simulink model "Asw_DCAC"  (R2023b)
settings: Solver=FixedStepDiscrete  StartTime=0.0  StopTime=inf  FixedStep=1e-8  RelTol=1e-3  EnableMultiTasking=on
undefined symbols (not defined in the file): f_Vref, Ts, V_DC
libraries: slpidlib x5, simulink x1
settings Model: Creator=VanillaC  LastModifiedBy=VanillaC
settings OptimizationCC: DefaultParameterBehavior=Inlined  EnhancedBackFolding=on  PassReuseOutputArgsAs=Individual arguments  ZeroExternalMemoryAtStartup=off  ZeroInternalMemoryAtStartup=off  MaxStackSize=64  OptimizeBlockOrder=speed  DifferentSizesBufferReuse=on  OptimizationCustomize=off  EfficientTunableParamExpr=on
settings DebuggingCC: ParameterTunabilityLossMsg=error
settings HardwareCC: ProdBitPerPointer=32  ProdBitPerSizeT=32  ProdBitPerPtrDiffT=32  ProdLargestAtomicInteger=Long  ProdLargestAtomicFloat=Double  ProdWordSize=32  ProdHWDeviceType=ARM Compatible->ARM Cortex-M
settings SFSimCC: MATLABDynamicMemAlloc=off
settings RTWCC: Description=Embedded Coder  SystemTargetFile=ert.tlc  GenCodeOnly=on  TemplateMakefile=ert_default_tmf  Toolchain=GNU Tools for ARM Embedded Processors
settings CodeAppCC: ForceParamTrailComments=on  IgnoreCustomStorageClasses=off  OperatorAnnotations=on  SimulinkDataObjDesc=on  SFDataObjDesc=on  InsertBlockDesc=on
settings ERTTargetCC: TargetLangStandard=C99 (ISO)  CodeReplacementLibrary=ARM Cortex-M  ExtModeTransport=3  ExtModeStaticAlloc=on  ExtModeStaticAllocSize=2048  ExtModeMexFile=ext_xcp  ExtModeIntrfLevel=Level2 - Open  InlinedParameterPlacement=NonHierarchical  ERTCustomFileTemplate=example_file_process.tlc

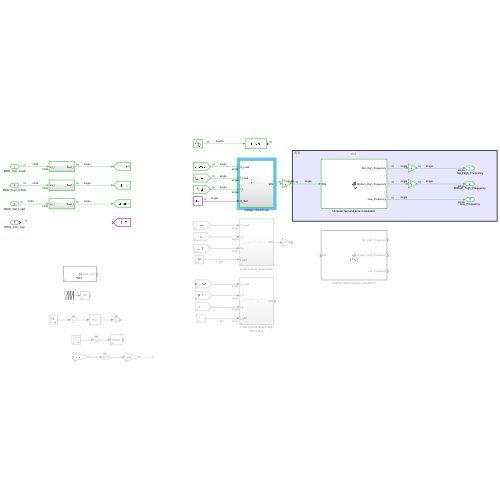
[thumbnail: Simulink's stored preview of the top-level diagram]
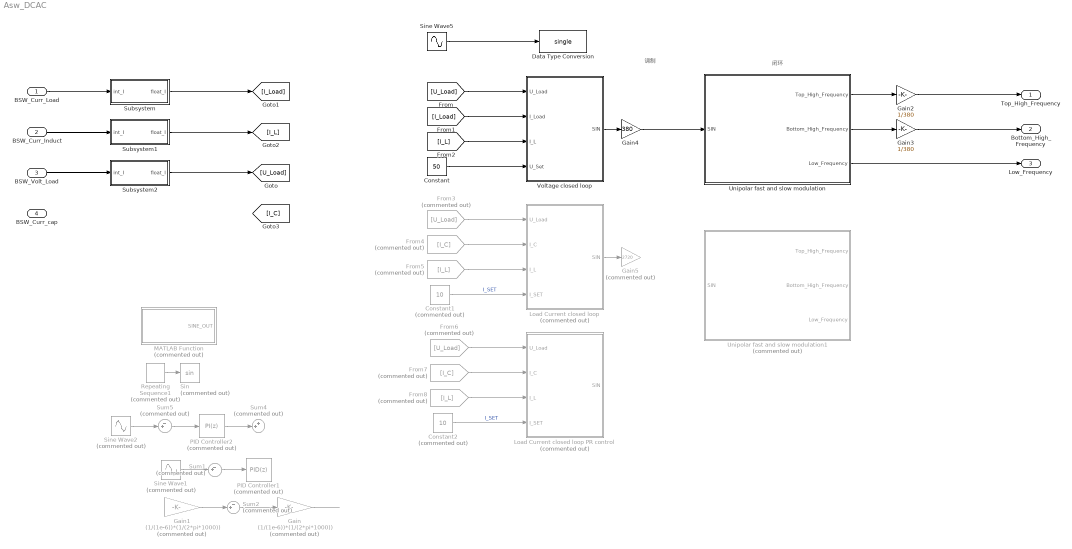
== system Asw_DCAC ==
  note: 闭环
  note: 调制
  BSW_Curr_Load : Inport  OutDataTypeStr=int32
  BSW_Curr_Induct : Inport  Port=2  OutDataTypeStr=int32
  BSW_Volt_Load : Inport  Port=3  OutDataTypeStr=int32
  BSW_Curr_cap : Inport  Port=4  OutDataTypeStr=single
  Constant : Constant  Value=50  OutDataTypeStr=single
  Constant1 : Constant  Commented=on  Value=10  OutDataTypeStr=single
  Constant2 : Constant  Commented=on  Value=10  OutDataTypeStr=single
  Data Type Conversion : DataTypeConversion  OutDataTypeStr=single  SaturateOnIntegerOverflow=off  RndMeth=Floor
  From3 : From  Commented=on  GotoTag=U_Load
  From4 : From  Commented=on  GotoTag=I_C
  From5 : From  Commented=on  GotoTag=I_L
  From6 : From  Commented=on  GotoTag=U_Load
  From7 : From  Commented=on  GotoTag=I_C
  From8 : From  Commented=on  GotoTag=I_L
  Gain : Gain  Commented=on  Gain=(1/(1e-6))*(1/(2*pi*1000))  OutDataTypeStr=single
  Gain1 : Gain  Commented=on  Gain=(1/(1e-6))*(1/(2*pi*1000))  OutDataTypeStr=single
  Gain2 : Gain  Gain=1/380
  Gain3 : Gain  Gain=1/380
  Gain4 : Gain  Gain=380
  Gain5 : Gain  Commented=on  Gain=2720
  Load Current closed loop : Subsystem  Commented=on
  Load Current closed loop PR control : Subsystem  Commented=on
  MATLAB Function : MATLAB Function  Commented=on  TreatAsAtomicUnit=on
  PID Controller1 : slpidlib/PID Controller  Commented=on  Controller=PID  Form=Parallel  TimeDomain=Discrete-time  UseExternalTs=off  SampleTime=-1  IntegratorMethod=Trapezoidal  FilterMethod=Forward Euler  ControllerParametersSource=internal  P=0.5  I=0.5  UseKiTs=off  D=0  N=100  UseFilter=off  TunerSelectOption=Transfer Function Based (PID Tuner App)  InitialConditionSource=internal  InitialConditionForIntegrator=0  InitialConditionForFilter=0  DifferentiatorICPrevScaledInput=0  ExternalReset=none  TrackingMode=off  Kt=1  LimitOutput=off  SatLimitsSource=internal  UpperSaturationLimit=inf  LowerSaturationLimit=-inf  LinearizeAsGain=on  AntiWindupMode=none  Kb=1  LimitIntegrator=off  UpperIntegratorSaturationLimit=inf  LowerIntegratorSaturationLimit=-inf  POutMin=[]  POutMax=[]  IOutMin=[]  IOutMax=[]  DOutMin=[]  DOutMax=[]  NOutMin=[]  NOutMax=[]  SumOutMin=[]  SumOutMax=[]  SaturationOutMin=[]  SaturationOutMax=[]  PParamMin=[]  PParamMax=[]  IParamMin=[]  IParamMax=[]  DParamMin=[]  DParamMax=[]  NParamMin=[]  NParamMax=[]  KbParamMin=[]  KbParamMax=[]  KtParamMin=[]  KtParamMax=[]  KbOutMin=[]  KbOutMax=[]  KtOutMin=[]  KtOutMax=[]  IntegratorOutMin=[]  IntegratorOutMax=[]  FilterOutMin=[]  FilterOutMax=[]  SumI1OutMin=[]  SumI1OutMax=[]  SumI2OutMin=[]  SumI2OutMax=[]  SumI3OutMin=[]  SumI3OutMax=[]  SumI4OutMin=[]  SumI4OutMax=[]  SumDOutMin=[]  SumDOutMax=[]  DifferentiatorOutMin=[]  DifferentiatorOutMax=[]  FilterDiffOutCoefMin=[]  FilterDiffOutCoefMax=[]  ReciprocalOutMin=[]  ReciprocalOutMax=[]  SumDenOutMin=[]  SumDenOutMax=[]  SumNumOutMin=[]  SumNumOutMax=[]  DivideOutMin=[]  DivideOutMax=[]  UdiffTsProdOutMin=[]  UdiffTsProdOutMax=[]  NTsProdOutMin=[]  NTsProdOutMax=[]  UintegralTsProdOutMin=[]  UintegralTsProdOutMax=[]  UngainTsProdOutMin=[]  UngainTsProdOutMax=[]  ClampingZeroOutDataTypeStr=Inherit: Inherit via back propagation  ClampingZeroOutMin=[]  ClampingZeroOutMax=[]  FilterDenConstantOutDataTypeStr=Inherit: Inherit via back propagation  FilterDenConstantOutMin=[]  FilterDenConstantOutMax=[]  PCopyOutDataTypeStr=Inherit: Inherit via back propagation  PCopyOutMin=[]  PCopyOutMax=[]  NCopyOutDataTypeStr=Inherit: Inherit via back propagation  NCopyOutMin=[]  NCopyOutMax=[]  IntegratorContinuousStateAttributes=''  IntegratorStateMustResolveToSignalObject=off  IntegratorRTWStateStorageClass=Auto  FilterContinuousStateAttributes=''  FilterStateMustResolveToSignalObject=off  FilterRTWStateStorageClass=Auto  ParallelPVariant=InternalParameters  IdealPVariant=Disabled  IVariant=InternalParameters  DVariant=InternalParameters  IntegratorVariant=Discrete  SatVariant=Disabled  AWVariant=Passthrough  PCopyVariant=Disabled  TRVariant=Disabled  FdbkBlocksVariant=Forward  IdealPFdbkVariant=Disabled  SatFdbkVariant=Disabled  DerivativeFilterVariant=Differentiator  NVariant=Passthrough  NCopyVariant=Disabled_SignalSpec  FilterICVariant=InternalICsDifferentiator  IntegratorICVariant=InternalICs  ExternalResetVariant=Disabled  TRSumVariant=Passthrough  SumFdbkVariant=Disabled  SumVariant=Sum_PID  TsampFilterVariant=InternalTs  TsampNgainVariant=Passthrough  TsampIntegralVariant=Disabled_SignalSpec  ExternalSaturationOutDataTypeStr=Inherit: Same as second input
  PID Controller2 : slpidlib/PID Controller  Commented=on  Controller=PI  Form=Parallel  TimeDomain=Discrete-time  UseExternalTs=off  SampleTime=-1  IntegratorMethod=Trapezoidal  FilterMethod=Forward Euler  ControllerParametersSource=internal  P=0.05115  I=30  UseKiTs=off  D=0  N=100  UseFilter=off  TunerSelectOption=Transfer Function Based (PID Tuner App)  InitialConditionSource=internal  InitialConditionForIntegrator=0  InitialConditionForFilter=0  DifferentiatorICPrevScaledInput=0  ExternalReset=none  TrackingMode=off  Kt=1  LimitOutput=off  SatLimitsSource=internal  UpperSaturationLimit=inf  LowerSaturationLimit=-inf  LinearizeAsGain=on  AntiWindupMode=none  Kb=1  LimitIntegrator=off  UpperIntegratorSaturationLimit=inf  LowerIntegratorSaturationLimit=-inf  POutMin=[]  POutMax=[]  IOutMin=[]  IOutMax=[]  DOutMin=[]  DOutMax=[]  NOutMin=[]  NOutMax=[]  SumOutMin=[]  SumOutMax=[]  SaturationOutMin=[]  SaturationOutMax=[]  PParamMin=[]  PParamMax=[]  IParamMin=[]  IParamMax=[]  DParamMin=[]  DParamMax=[]  NParamMin=[]  NParamMax=[]  KbParamMin=[]  KbParamMax=[]  KtParamMin=[]  KtParamMax=[]  KbOutMin=[]  KbOutMax=[]  KtOutMin=[]  KtOutMax=[]  IntegratorOutMin=[]  IntegratorOutMax=[]  FilterOutMin=[]  FilterOutMax=[]  SumI1OutMin=[]  SumI1OutMax=[]  SumI2OutMin=[]  SumI2OutMax=[]  SumI3OutMin=[]  SumI3OutMax=[]  SumI4OutMin=[]  SumI4OutMax=[]  SumDOutMin=[]  SumDOutMax=[]  DifferentiatorOutMin=[]  DifferentiatorOutMax=[]  FilterDiffOutCoefMin=[]  FilterDiffOutCoefMax=[]  ReciprocalOutMin=[]  ReciprocalOutMax=[]  SumDenOutMin=[]  SumDenOutMax=[]  SumNumOutMin=[]  SumNumOutMax=[]  DivideOutMin=[]  DivideOutMax=[]  UdiffTsProdOutMin=[]  UdiffTsProdOutMax=[]  NTsProdOutMin=[]  NTsProdOutMax=[]  UintegralTsProdOutMin=[]  UintegralTsProdOutMax=[]  UngainTsProdOutMin=[]  UngainTsProdOutMax=[]  ClampingZeroOutDataTypeStr=Inherit: Inherit via back propagation  ClampingZeroOutMin=[]  ClampingZeroOutMax=[]  FilterDenConstantOutDataTypeStr=Inherit: Inherit via back propagation  FilterDenConstantOutMin=[]  FilterDenConstantOutMax=[]  PCopyOutDataTypeStr=Inherit: Inherit via back propagation  PCopyOutMin=[]  PCopyOutMax=[]  NCopyOutDataTypeStr=Inherit: Inherit via back propagation  NCopyOutMin=[]  NCopyOutMax=[]  IntegratorContinuousStateAttributes=''  IntegratorStateMustResolveToSignalObject=off  IntegratorRTWStateStorageClass=Auto  FilterContinuousStateAttributes=''  FilterStateMustResolveToSignalObject=off  FilterRTWStateStorageClass=Auto  ParallelPVariant=InternalParameters  IdealPVariant=Disabled  IVariant=InternalParameters  DVariant=Disabled  IntegratorVariant=Discrete  SatVariant=Disabled  AWVariant=Passthrough  PCopyVariant=Disabled  TRVariant=Disabled  FdbkBlocksVariant=Forward  IdealPFdbkVariant=Disabled  SatFdbkVariant=Disabled  DerivativeFilterVariant=Disabled  NVariant=Disabled  NCopyVariant=Disabled_SignalSpec  FilterICVariant=Disabled  IntegratorICVariant=InternalICs  ExternalResetVariant=Disabled  TRSumVariant=Passthrough  SumFdbkVariant=Disabled  SumVariant=Sum_PI  TsampFilterVariant=InternalTs  TsampNgainVariant=Passthrough  TsampIntegralVariant=Disabled_SignalSpec  ExternalSaturationOutDataTypeStr=Inherit: Same as second input
  Repeating Sequence1 : simulink/Sources/Repeating Sequence  Commented=on  rep_seq_t=[0 1/1000]  rep_seq_y=[0 2*pi]
  Sin : Trigonometry  Commented=on
  Sine Wave1 : Sin  Commented=on  Frequency=2*pi*1000  SampleTime=Ts
  Sine Wave2 : Sin  Commented=on  Amplitude=311  Frequency=f_Vref  SampleTime=Ts
  Sine Wave5 : Sin  Frequency=2*pi*1000  SampleTime=Ts
  Subsystem : Subsystem
  Subsystem1 : Subsystem
  Subsystem2 : Subsystem
  Sum1 : Sum  Commented=on  Inputs=-+|  OutDataTypeStr=single
  Sum2 : Sum  Commented=on  Inputs=-+|  OutDataTypeStr=single
  Sum4 : Sum  Commented=on  Inputs=++|
  Sum5 : Sum  Commented=on  Inputs=-+|  OutDataTypeStr=single
  Unipolar fast and slow modulation : MATLAB Function  TreatAsAtomicUnit=on
  Unipolar fast and slow modulation1 : MATLAB Function  Commented=on  TreatAsAtomicUnit=on
  Voltage closed loop : Subsystem
  Top_High_Frequency : Outport  OutDataTypeStr=single
  Bottom_High_Frequency : Outport  Port=2  OutDataTypeStr=single
  Low_Frequency : Outport  Port=3  OutDataTypeStr=single
  wires:
  Unipolar fast and slow modulation/2(Bottom_High_Frequency) -> Gain3/1
  Unipolar fast and slow modulation/1(Top_High_Frequency) -> Gain2/1
  Sum5/1 -> PID Controller2/1
  Sine Wave1/1 -> Sum1/2
  Sum1/1 -> PID Controller1/1
  Sine Wave5/1 -> Data Type Conversion/1
  Gain/1 -> ?
  Gain1/1 -> Sum2/2
  Sum2/1 -> Gain/1
  Sine Wave2/1 -> Sum5/2
  PID Controller2/1 -> Sum4/2
  Repeating Sequence1/1 -> Sin/1
  Constant/1 -> Voltage closed loop/4(U_Set)
  Constant1/1 -> Load Current closed loop/4(I_SET)  "I_SET"
  From5/1 -> Load Current closed loop/3(I_L)
  From4/1 -> Load Current closed loop/2(I_C)
  From3/1 -> Load Current closed loop/1(U_Load)
  [U_Load] -> Voltage closed loop/1(U_Load)
  [I_Load] -> Voltage closed loop/2(I_Load)
  [I_L] -> Voltage closed loop/3(I_L)
  From7/1 -> Load Current closed loop PR control/2(I_C)
  Constant2/1 -> Load Current closed loop PR control/4(I_SET)  "I_SET"
  From6/1 -> Load Current closed loop PR control/1(U_Load)
  From8/1 -> Load Current closed loop PR control/3(I_L)
  Gain2/1 -> Top_High_Frequency/1
  Gain3/1 -> Bottom_High_Frequency/1
  Unipolar fast and slow modulation/3(Low_Frequency) -> Low_Frequency/1
  Load Current closed loop/1(SIN) -> Gain5/1
  BSW_Curr_Load/1 -> Subsystem/1(int_I)
  BSW_Curr_Induct/1 -> Subsystem1/1(int_I)
  BSW_Volt_Load/1 -> Subsystem2/1(int_I)
  Subsystem/1(float_I) -> [I_Load]
  Subsystem1/1(float_I) -> [I_L]
  Subsystem2/1(float_I) -> [U_Load]
  Gain4/1 -> Unipolar fast and slow modulation/1(SIN)
  Voltage closed loop/1(SIN) -> Gain4/1

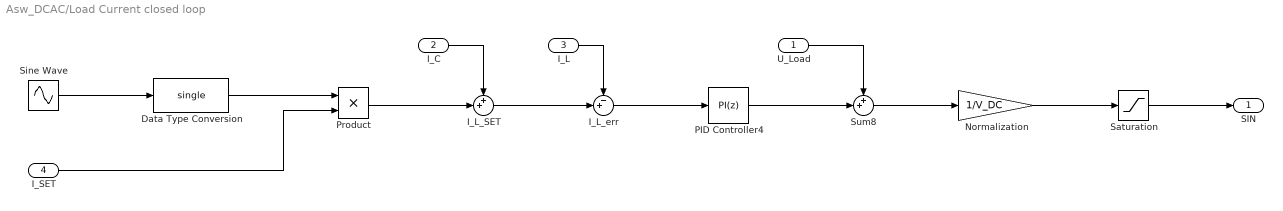
== system Asw_DCAC/Load Current closed loop ==
  U_Load : Inport  OutDataTypeStr=single
  I_C : Inport  Port=2  OutDataTypeStr=single
  I_L : Inport  Port=3  OutDataTypeStr=single
  I_SET : Inport  Port=4
  Data Type Conversion : DataTypeConversion  OutDataTypeStr=single  SaturateOnIntegerOverflow=off  RndMeth=Floor
  I_L_SET : Sum  Inputs=++|  OutDataTypeStr=single
  I_L_err : Sum  Inputs=-+|  OutDataTypeStr=single
  Normalization : Gain  Gain=1/V_DC  OutDataTypeStr=single
  PID Controller4 : slpidlib/PID Controller  Controller=PI  Form=Parallel  TimeDomain=Discrete-time  UseExternalTs=off  SampleTime=Ts  IntegratorMethod=Trapezoidal  FilterMethod=Forward Euler  ControllerParametersSource=internal  P=5  I=1  UseKiTs=off  D=0  N=100  UseFilter=off  TunerSelectOption=Transfer Function Based (PID Tuner App)  InitialConditionSource=internal  InitialConditionForIntegrator=0  InitialConditionForFilter=0  DifferentiatorICPrevScaledInput=0  ExternalReset=none  TrackingMode=off  Kt=1  LimitOutput=off  SatLimitsSource=internal  UpperSaturationLimit=inf  LowerSaturationLimit=-inf  LinearizeAsGain=on  AntiWindupMode=none  Kb=1  LimitIntegrator=off  UpperIntegratorSaturationLimit=inf  LowerIntegratorSaturationLimit=-inf  POutMin=[]  POutMax=[]  IOutMin=[]  IOutMax=[]  DOutMin=[]  DOutMax=[]  NOutMin=[]  NOutMax=[]  SumOutMin=[]  SumOutMax=[]  SaturationOutMin=[]  SaturationOutMax=[]  PParamMin=[]  PParamMax=[]  IParamMin=[]  IParamMax=[]  DParamMin=[]  DParamMax=[]  NParamMin=[]  NParamMax=[]  KbParamMin=[]  KbParamMax=[]  KtParamMin=[]  KtParamMax=[]  KbOutMin=[]  KbOutMax=[]  KtOutMin=[]  KtOutMax=[]  IntegratorOutMin=[]  IntegratorOutMax=[]  FilterOutMin=[]  FilterOutMax=[]  SumI1OutMin=[]  SumI1OutMax=[]  SumI2OutMin=[]  SumI2OutMax=[]  SumI3OutMin=[]  SumI3OutMax=[]  SumI4OutMin=[]  SumI4OutMax=[]  SumDOutMin=[]  SumDOutMax=[]  DifferentiatorOutMin=[]  DifferentiatorOutMax=[]  FilterDiffOutCoefMin=[]  FilterDiffOutCoefMax=[]  ReciprocalOutMin=[]  ReciprocalOutMax=[]  SumDenOutMin=[]  SumDenOutMax=[]  SumNumOutMin=[]  SumNumOutMax=[]  DivideOutMin=[]  DivideOutMax=[]  UdiffTsProdOutMin=[]  UdiffTsProdOutMax=[]  NTsProdOutMin=[]  NTsProdOutMax=[]  UintegralTsProdOutMin=[]  UintegralTsProdOutMax=[]  UngainTsProdOutMin=[]  UngainTsProdOutMax=[]  ClampingZeroOutDataTypeStr=Inherit: Inherit via back propagation  ClampingZeroOutMin=[]  ClampingZeroOutMax=[]  FilterDenConstantOutDataTypeStr=Inherit: Inherit via back propagation  FilterDenConstantOutMin=[]  FilterDenConstantOutMax=[]  PCopyOutDataTypeStr=Inherit: Inherit via back propagation  PCopyOutMin=[]  PCopyOutMax=[]  NCopyOutDataTypeStr=Inherit: Inherit via back propagation  NCopyOutMin=[]  NCopyOutMax=[]  IntegratorContinuousStateAttributes=''  IntegratorStateMustResolveToSignalObject=off  IntegratorRTWStateStorageClass=Auto  FilterContinuousStateAttributes=''  FilterStateMustResolveToSignalObject=off  FilterRTWStateStorageClass=Auto  ParallelPVariant=InternalParameters  IdealPVariant=Disabled  IVariant=InternalParameters  DVariant=Disabled  IntegratorVariant=Discrete  SatVariant=Disabled  AWVariant=Passthrough  PCopyVariant=Disabled  TRVariant=Disabled  FdbkBlocksVariant=Forward  IdealPFdbkVariant=Disabled  SatFdbkVariant=Disabled  DerivativeFilterVariant=Disabled  NVariant=Disabled  NCopyVariant=Disabled_SignalSpec  FilterICVariant=Disabled  IntegratorICVariant=InternalICs  ExternalResetVariant=Disabled  TRSumVariant=Passthrough  SumFdbkVariant=Disabled  SumVariant=Sum_PI  TsampFilterVariant=InternalTs  TsampNgainVariant=Passthrough  TsampIntegralVariant=Disabled_SignalSpec  ExternalSaturationOutDataTypeStr=Inherit: Same as second input
  Product : Product  OutDataTypeStr=single
  Saturation : Saturate  UpperLimit=1  LowerLimit=-1  OutDataTypeStr=single
  Sine Wave : Sin  Frequency=2*pi*1000  SampleTime=Ts
  Sum8 : Sum  Inputs=++|  OutDataTypeStr=single
  SIN : Outport
  wires:
  I_L_err/1 -> PID Controller4/1
  PID Controller4/1 -> Sum8/2
  Sine Wave/1 -> Data Type Conversion/1
  Data Type Conversion/1 -> Product/1
  I_L/1 -> I_L_err/1
  Sum8/1 -> Normalization/1
  Saturation/1 -> SIN/1
  I_SET/1 -> Product/2
  Normalization/1 -> Saturation/1
  U_Load/1 -> Sum8/1
  Product/1 -> I_L_SET/2
  I_L_SET/1 -> I_L_err/2
  I_C/1 -> I_L_SET/1

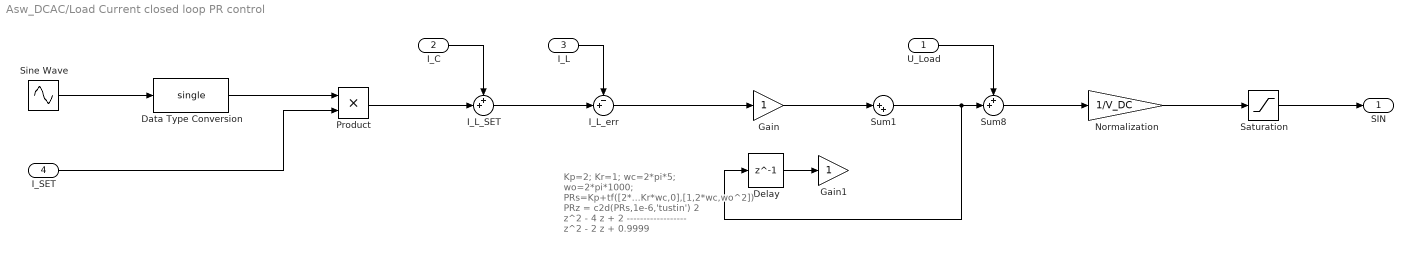
== system Asw_DCAC/Load Current closed loop PR control ==
  note: Kp=2; Kr=1; wc=2*pi*5; wo=2*pi*1000; PRs=Kp+tf([2*Kr*wc,0],[1,2*wc,wo^2]) PRz = c2d(PRs,1e-6,'tustin')
      |
      |  2 z^2 - 4 z + 2
      |   ------------------
      |   z^2 - 2 z + 0.9999
  U_Load : Inport  OutDataTypeStr=single
  I_C : Inport  Port=2  OutDataTypeStr=single
  I_L : Inport  Port=3  OutDataTypeStr=single
  I_SET : Inport  Port=4  OutDataTypeStr=single
  Data Type Conversion : DataTypeConversion  OutDataTypeStr=single  SaturateOnIntegerOverflow=off  RndMeth=Floor
  Delay : Delay  DelayLength=1
  Gain : Gain  OutDataTypeStr=single
  Gain1 : Gain  OutDataTypeStr=single
  I_L_SET : Sum  Inputs=++|  OutDataTypeStr=single
  I_L_err : Sum  Inputs=-+|  OutDataTypeStr=single
  Normalization : Gain  Gain=1/V_DC  OutDataTypeStr=single
  Product : Product  OutDataTypeStr=single
  Saturation : Saturate  UpperLimit=1  LowerLimit=-1  OutDataTypeStr=single
  Sine Wave : Sin  Frequency=2*pi*1000  SampleTime=Ts
  Sum1 : Sum  Inputs=|++  OutDataTypeStr=single
  Sum8 : Sum  Inputs=++|  OutDataTypeStr=single
  SIN : Outport
  wires:
  Sine Wave/1 -> Data Type Conversion/1
  Data Type Conversion/1 -> Product/1
  I_L/1 -> I_L_err/1
  Sum8/1 -> Normalization/1
  Saturation/1 -> SIN/1
  I_SET/1 -> Product/2
  Normalization/1 -> Saturation/1
  U_Load/1 -> Sum8/1
  Product/1 -> I_L_SET/2
  I_L_SET/1 -> I_L_err/2
  I_C/1 -> I_L_SET/1
  Gain/1 -> Sum1/1
  Delay/1 -> Gain1/1
  Sum1/1 -> Delay/1, Sum8/2
  I_L_err/1 -> Gain/1

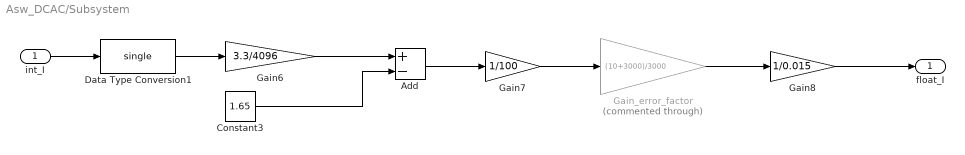
== system Asw_DCAC/Subsystem ==
  int_I : Inport  OutDataTypeStr=int32
  Add : Sum  Inputs=+-  OutDataTypeStr=single
  Constant3 : Constant  Value=1.65  OutDataTypeStr=single  SampleTime=-1
  Data Type Conversion1 : DataTypeConversion  OutDataTypeStr=single  SaturateOnIntegerOverflow=off  RndMeth=Floor
  Gain6 : Gain  Gain=3.3/4096  OutDataTypeStr=single
  Gain7 : Gain  Gain=1/100  OutDataTypeStr=single
  Gain8 : Gain  Gain=1/0.015  OutDataTypeStr=single
  Gain_error_factor : Gain  Commented=through  Gain=(10+3000)/3000  OutDataTypeStr=single
  float_I : Outport
  wires:
  Gain_error_factor/1 -> Gain8/1
  Constant3/1 -> Add/2
  Gain6/1 -> Add/1
  Gain7/1 -> Gain_error_factor/1
  Gain8/1 -> float_I/1
  int_I/1 -> Data Type Conversion1/1
  Data Type Conversion1/1 -> Gain6/1
  Add/1 -> Gain7/1

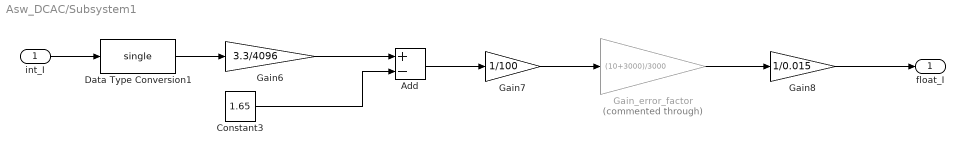
== system Asw_DCAC/Subsystem1 ==
  int_I : Inport  OutDataTypeStr=int32
  Add : Sum  Inputs=+-  OutDataTypeStr=single
  Constant3 : Constant  Value=1.65  OutDataTypeStr=single  SampleTime=-1
  Data Type Conversion1 : DataTypeConversion  OutDataTypeStr=single  SaturateOnIntegerOverflow=off  RndMeth=Floor
  Gain6 : Gain  Gain=3.3/4096  OutDataTypeStr=single
  Gain7 : Gain  Gain=1/100  OutDataTypeStr=single
  Gain8 : Gain  Gain=1/0.015  OutDataTypeStr=single
  Gain_error_factor : Gain  Commented=through  Gain=(10+3000)/3000  OutDataTypeStr=single
  float_I : Outport
  wires:
  Add/1 -> Gain7/1
  Data Type Conversion1/1 -> Gain6/1
  int_I/1 -> Data Type Conversion1/1
  Gain8/1 -> float_I/1
  Gain7/1 -> Gain_error_factor/1
  Gain6/1 -> Add/1
  Constant3/1 -> Add/2
  Gain_error_factor/1 -> Gain8/1

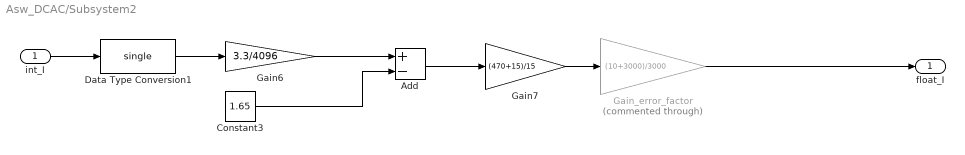
== system Asw_DCAC/Subsystem2 ==
  int_I : Inport  OutDataTypeStr=int32
  Add : Sum  Inputs=+-  OutDataTypeStr=single
  Constant3 : Constant  Value=1.65  OutDataTypeStr=single  SampleTime=-1
  Data Type Conversion1 : DataTypeConversion  OutDataTypeStr=single  SaturateOnIntegerOverflow=off  RndMeth=Floor
  Gain6 : Gain  Gain=3.3/4096  OutDataTypeStr=single
  Gain7 : Gain  Gain=(470+15)/15  OutDataTypeStr=single
  Gain_error_factor : Gain  Commented=through  Gain=(10+3000)/3000  OutDataTypeStr=single
  float_I : Outport
  wires:
  Constant3/1 -> Add/2
  Gain6/1 -> Add/1
  Gain7/1 -> Gain_error_factor/1
  Gain_error_factor/1 -> float_I/1
  int_I/1 -> Data Type Conversion1/1
  Data Type Conversion1/1 -> Gain6/1
  Add/1 -> Gain7/1

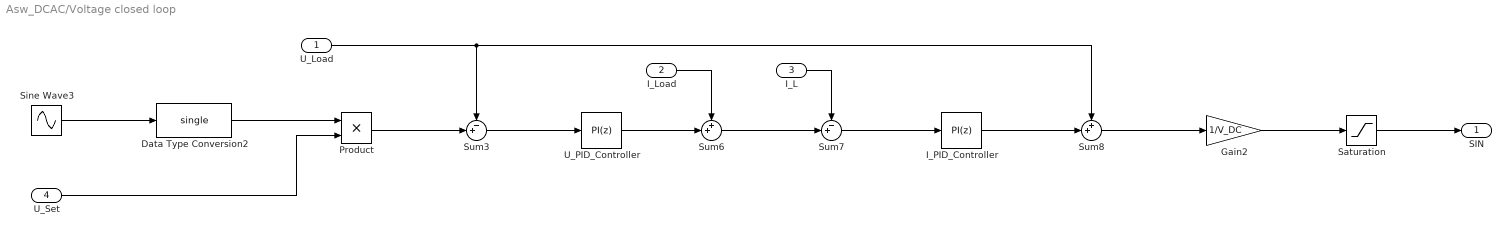
== system Asw_DCAC/Voltage closed loop ==
  U_Load : Inport  OutDataTypeStr=single
  I_Load : Inport  Port=2  OutDataTypeStr=single
  I_L : Inport  Port=3  OutDataTypeStr=single
  U_Set : Inport  Port=4
  Data Type Conversion2 : DataTypeConversion  OutDataTypeStr=single  SaturateOnIntegerOverflow=off  RndMeth=Floor
  Gain2 : Gain  Gain=1/V_DC  OutDataTypeStr=single
  I_PID_Controller : slpidlib/PID Controller  Controller=PI  Form=Parallel  TimeDomain=Discrete-time  UseExternalTs=off  SampleTime=Ts  IntegratorMethod=Trapezoidal  FilterMethod=Forward Euler  ControllerParametersSource=internal  P=1.6  I=0.0001  UseKiTs=off  D=0  N=100  UseFilter=off  TunerSelectOption=Transfer Function Based (PID Tuner App)  InitialConditionSource=internal  InitialConditionForIntegrator=0  InitialConditionForFilter=0  DifferentiatorICPrevScaledInput=0  ExternalReset=none  TrackingMode=off  Kt=1  LimitOutput=off  SatLimitsSource=internal  UpperSaturationLimit=inf  LowerSaturationLimit=-inf  LinearizeAsGain=on  AntiWindupMode=none  Kb=1  LimitIntegrator=off  UpperIntegratorSaturationLimit=inf  LowerIntegratorSaturationLimit=-inf  POutMin=[]  POutMax=[]  IOutMin=[]  IOutMax=[]  DOutMin=[]  DOutMax=[]  NOutMin=[]  NOutMax=[]  SumOutMin=[]  SumOutMax=[]  SaturationOutMin=[]  SaturationOutMax=[]  PParamMin=[]  PParamMax=[]  IParamMin=[]  IParamMax=[]  DParamMin=[]  DParamMax=[]  NParamMin=[]  NParamMax=[]  KbParamMin=[]  KbParamMax=[]  KtParamMin=[]  KtParamMax=[]  KbOutMin=[]  KbOutMax=[]  KtOutMin=[]  KtOutMax=[]  IntegratorOutMin=[]  IntegratorOutMax=[]  FilterOutMin=[]  FilterOutMax=[]  SumI1OutMin=[]  SumI1OutMax=[]  SumI2OutMin=[]  SumI2OutMax=[]  SumI3OutMin=[]  SumI3OutMax=[]  SumI4OutMin=[]  SumI4OutMax=[]  SumDOutMin=[]  SumDOutMax=[]  DifferentiatorOutMin=[]  DifferentiatorOutMax=[]  FilterDiffOutCoefMin=[]  FilterDiffOutCoefMax=[]  ReciprocalOutMin=[]  ReciprocalOutMax=[]  SumDenOutMin=[]  SumDenOutMax=[]  SumNumOutMin=[]  SumNumOutMax=[]  DivideOutMin=[]  DivideOutMax=[]  UdiffTsProdOutMin=[]  UdiffTsProdOutMax=[]  NTsProdOutMin=[]  NTsProdOutMax=[]  UintegralTsProdOutMin=[]  UintegralTsProdOutMax=[]  UngainTsProdOutMin=[]  UngainTsProdOutMax=[]  ClampingZeroOutDataTypeStr=Inherit: Inherit via back propagation  ClampingZeroOutMin=[]  ClampingZeroOutMax=[]  FilterDenConstantOutDataTypeStr=Inherit: Inherit via back propagation  FilterDenConstantOutMin=[]  FilterDenConstantOutMax=[]  PCopyOutDataTypeStr=Inherit: Inherit via back propagation  PCopyOutMin=[]  PCopyOutMax=[]  NCopyOutDataTypeStr=Inherit: Inherit via back propagation  NCopyOutMin=[]  NCopyOutMax=[]  IntegratorContinuousStateAttributes=''  IntegratorStateMustResolveToSignalObject=off  IntegratorRTWStateStorageClass=Auto  FilterContinuousStateAttributes=''  FilterStateMustResolveToSignalObject=off  FilterRTWStateStorageClass=Auto  ParallelPVariant=InternalParameters  IdealPVariant=Disabled  IVariant=InternalParameters  DVariant=Disabled  IntegratorVariant=Discrete  SatVariant=Disabled  AWVariant=Passthrough  PCopyVariant=Disabled  TRVariant=Disabled  FdbkBlocksVariant=Forward  IdealPFdbkVariant=Disabled  SatFdbkVariant=Disabled  DerivativeFilterVariant=Disabled  NVariant=Disabled  NCopyVariant=Disabled_SignalSpec  FilterICVariant=Disabled  IntegratorICVariant=InternalICs  ExternalResetVariant=Disabled  TRSumVariant=Passthrough  SumFdbkVariant=Disabled  SumVariant=Sum_PI  TsampFilterVariant=InternalTs  TsampNgainVariant=Passthrough  TsampIntegralVariant=Disabled_SignalSpec  ExternalSaturationOutDataTypeStr=Inherit: Same as second input
  Product : Product  OutDataTypeStr=single
  Saturation : Saturate  UpperLimit=1  LowerLimit=-1  OutDataTypeStr=single
  Sine Wave3 : Sin  Frequency=2*pi*1000  SampleTime=Ts
  Sum3 : Sum  Inputs=-+|  OutDataTypeStr=single
  Sum6 : Sum  Inputs=++|  OutDataTypeStr=single
  Sum7 : Sum  Inputs=-+|  OutDataTypeStr=single
  Sum8 : Sum  Inputs=++|  OutDataTypeStr=single
  U_PID_Controller : slpidlib/PID Controller  Controller=PI  Form=Parallel  TimeDomain=Discrete-time  UseExternalTs=off  SampleTime=Ts  IntegratorMethod=Trapezoidal  FilterMethod=Forward Euler  ControllerParametersSource=internal  P=1  I=0.0001  UseKiTs=off  D=0  N=100  UseFilter=on  TunerSelectOption=Transfer Function Based (PID Tuner App)  InitialConditionSource=internal  InitialConditionForIntegrator=0  InitialConditionForFilter=0  DifferentiatorICPrevScaledInput=0  ExternalReset=none  TrackingMode=off  Kt=1  LimitOutput=off  SatLimitsSource=internal  UpperSaturationLimit=inf  LowerSaturationLimit=-inf  LinearizeAsGain=on  AntiWindupMode=none  Kb=1  LimitIntegrator=off  UpperIntegratorSaturationLimit=inf  LowerIntegratorSaturationLimit=-inf  POutMin=[]  POutMax=[]  IOutMin=[]  IOutMax=[]  DOutMin=[]  DOutMax=[]  NOutMin=[]  NOutMax=[]  SumOutMin=[]  SumOutMax=[]  SaturationOutMin=[]  SaturationOutMax=[]  PParamMin=[]  PParamMax=[]  IParamMin=[]  IParamMax=[]  DParamMin=[]  DParamMax=[]  NParamMin=[]  NParamMax=[]  KbParamMin=[]  KbParamMax=[]  KtParamMin=[]  KtParamMax=[]  KbOutMin=[]  KbOutMax=[]  KtOutMin=[]  KtOutMax=[]  IntegratorOutMin=[]  IntegratorOutMax=[]  FilterOutMin=[]  FilterOutMax=[]  SumI1OutMin=[]  SumI1OutMax=[]  SumI2OutMin=[]  SumI2OutMax=[]  SumI3OutMin=[]  SumI3OutMax=[]  SumI4OutMin=[]  SumI4OutMax=[]  SumDOutMin=[]  SumDOutMax=[]  DifferentiatorOutMin=[]  DifferentiatorOutMax=[]  FilterDiffOutCoefMin=[]  FilterDiffOutCoefMax=[]  ReciprocalOutMin=[]  ReciprocalOutMax=[]  SumDenOutMin=[]  SumDenOutMax=[]  SumNumOutMin=[]  SumNumOutMax=[]  DivideOutMin=[]  DivideOutMax=[]  UdiffTsProdOutMin=[]  UdiffTsProdOutMax=[]  NTsProdOutMin=[]  NTsProdOutMax=[]  UintegralTsProdOutMin=[]  UintegralTsProdOutMax=[]  UngainTsProdOutMin=[]  UngainTsProdOutMax=[]  ClampingZeroOutDataTypeStr=Inherit: Inherit via back propagation  ClampingZeroOutMin=[]  ClampingZeroOutMax=[]  FilterDenConstantOutDataTypeStr=Inherit: Inherit via back propagation  FilterDenConstantOutMin=[]  FilterDenConstantOutMax=[]  PCopyOutDataTypeStr=Inherit: Inherit via back propagation  PCopyOutMin=[]  PCopyOutMax=[]  NCopyOutDataTypeStr=Inherit: Inherit via back propagation  NCopyOutMin=[]  NCopyOutMax=[]  IntegratorContinuousStateAttributes=''  IntegratorStateMustResolveToSignalObject=off  IntegratorRTWStateStorageClass=Auto  FilterContinuousStateAttributes=''  FilterStateMustResolveToSignalObject=off  FilterRTWStateStorageClass=Auto  ParallelPVariant=InternalParameters  IdealPVariant=Disabled  IVariant=InternalParameters  DVariant=Disabled  IntegratorVariant=Discrete  SatVariant=Disabled  AWVariant=Passthrough  PCopyVariant=Disabled  TRVariant=Disabled  FdbkBlocksVariant=Forward  IdealPFdbkVariant=Disabled  SatFdbkVariant=Disabled  DerivativeFilterVariant=Disabled  NVariant=Disabled  NCopyVariant=Disabled_SignalSpec  FilterICVariant=Disabled  IntegratorICVariant=InternalICs  ExternalResetVariant=Disabled  TRSumVariant=Passthrough  SumFdbkVariant=Disabled  SumVariant=Sum_PI  TsampFilterVariant=InternalTs  TsampNgainVariant=Passthrough  TsampIntegralVariant=Disabled_SignalSpec  ExternalSaturationOutDataTypeStr=Inherit: Same as second input
  SIN : Outport
  wires:
  U_Load/1 -> Sum8/1, Sum3/1
  Gain2/1 -> Saturation/1
  Sum6/1 -> Sum7/2
  U_Set/1 -> Product/2
  Sum3/1 -> U_PID_Controller/1
  I_Load/1 -> Sum6/1
  Saturation/1 -> SIN/1
  U_PID_Controller/1 -> Sum6/2
  Sum8/1 -> Gain2/1
  I_L/1 -> Sum7/1
  Data Type Conversion2/1 -> Product/1
  Sine Wave3/1 -> Data Type Conversion2/1
  Product/1 -> Sum3/2
  I_PID_Controller/1 -> Sum8/2
  Sum7/1 -> I_PID_Controller/1

== matlab function Asw_DCAC/Unipolar fast and slow modulation1 ==
  data: SIN input single; Top_High_Frequency output single; Bottom_High_Frequency output single; Low_Frequency output single
function [Top_High_Frequency, Bottom_High_Frequency, Low_Frequency]  = SPWM(SIN)
    
    Top_High_Frequency = single(0);
    Bottom_High_Frequency = single(0);
    Low_Frequency = single(0);
    
    if (SIN >= 0)
        Top_High_Frequency = SIN;
        Low_Frequency = single(0);
    else
        Bottom_High_Frequency = -SIN;
        Low_Frequency = single(1);
    end

  % persistent Dui;
  % persistent Qui;
  % 
  % if isempty(Dui)
  %   Dui = single(0);
  %   Qui = single(0);
  % end
  % 
  % Iderr = Idcmd - Idfbk;
  % Dup = DCurKp * Iderr;
  % Dui = Dui + DCurKi * Iderr * Ts;
  % 
  % Udcmd = Dup + Dui - we * Lq * Iqfbk;
  % 
  % Iqerr = Iqcmd - Iqfbk;
  % Qup = QCurKp * Iqerr;
  % Qui = Qui + QCurKi * Iqerr * Ts;
  % 
  % Uqcmd = Qup + Qui + we * Ld *Idfbk;

end

== matlab function Asw_DCAC/MATLAB Function ==
  data: SINE_OUT output single
function SINE_OUT = SINE()

    persistent SINE;      
    persistent flag;
    persistent add;
    SINE_OUT = single(0);
    if(isempty(flag))
        SINE = [0	0.0062831440	0.012566040	0.018848440	0.025130095	0.031410757	0.037690181	0.043968119	0.050244316	0.056518536	0.062790520	0.069060028	0.075326808	0.081590615	0.087851197	0.094108313	0.10036171	0.10661115	0.11285639	0.11909716	0.12533323	0.13156436	0.13779029	0.14401078	0.15022559	0.15643446	0.16263716	0.16883345	0.17502306	0.18120576	0.18738131	0.19354947	0.19970998	0.20586261	0.21200711	0.21814324	0.22427076	0.23038943	0.23649900	0.24259923	0.24868989	0.25477073	0.26084152	0.26690200	0.27295193	0.27899110	0.28501925	0.29103616	0.29704159	0.30303526	0.30901700	0.31498653	0.32094362	0.32688802	0.33281955	0.33873793	0.34464294	0.35053432	0.35641187	0.36227536	0.36812454	0.37395921	0.37977910	0.38558400	0.39137366	0.39714789	0.40290645	0.40864909	0.41437557	0.42008573	0.42577928	0.43145606	0.43711576	0.44275823	0.44838321	0.45399049	0.45957986	0.46515107	0.47070393	0.47623819	0.48175368	0.48725012	0.49272734	0.49818510	0.50362319	0.50904143	0.51443952	0.51981735	0.52517462	0.53051120	0.53582680	0.54112124	0.54639435	0.55164587	0.55687565	0.56208336	0.56726897	0.57243210	0.57757270	0.58269048	0.58778524	0.59285682	0.59790498	0.60292953	0.60793030	0.61290705	0.61785960	0.62278777	0.62769139	0.63257015	0.63742399	0.64225262	0.64705598	0.65183371	0.65658575	0.66131186	0.66601187	0.67068559	0.67533278	0.67995340	0.68454713	0.68911380	0.69365329	0.69816542	0.70264995	0.70710677	0.71153569	0.71593648	0.72030902	0.72465312	0.72896862	0.73325533	0.73751312	0.74174178	0.74594116	0.75011104	0.75425136	0.75836194	0.76244253	0.76649302	0.77051324	0.77450305	0.77846229	0.78239083	0.78628844	0.79015499	0.79399037	0.79779446	0.80156696	0.80530787	0.80901700	0.81269419	0.81633925	0.81995213	0.82353258	0.82708055	0.83059591	0.83407843	0.83752805	0.84094459	0.84432793	0.84767795	0.85099447	0.85427743	0.85752666	0.86074203	0.86392343	0.86707067	0.87018377	0.87326247	0.87630665	0.87931633	0.88229120	0.88523132	0.88813645	0.89100653	0.89384145	0.89664102	0.89940524	0.90213394	0.90482706	0.90748441	0.91010594	0.91269159	0.91524118	0.91775465	0.92023182	0.92267275	0.92507720	0.92744517	0.92977649	0.93207109	0.93432891	0.93654990	0.93873388	0.94088078	0.94299054	0.94506305	0.94709831	0.94909614	0.95105654	0.95297933	0.95486456	0.95671207	0.95852178	0.96029371	0.96202767	0.96372366	0.96538162	0.96700150	0.96858317	0.97012657	0.97163171	0.97309852	0.97452688	0.97591674	0.97726810	0.97858089	0.97985506	0.98109055	0.98228723	0.98344523	0.98456436	0.98564458	0.98668593	0.98768836	0.98865175	0.98957610	0.99046141	0.99130762	0.99211472	0.99288261	0.99361134	0.99430078	0.99495101	0.99556196	0.99613363	0.99666595	0.99715889	0.99761254	0.99802673	0.99840152	0.99873698	0.99903291	0.99928945	0.99950653	0.99968421	0.99982238	0.99992102	0.99998027	1	0.99998027	0.99992102	0.99982238	0.99968421	0.99950653	0.99928945	0.99903291	0.99873698	0.99840152	0.99802673	0.99761254	0.99715889	0.99666595	0.99613363	0.99556196	0.99495101	0.99430078	0.99361134	0.99288261	0.99211472	0.99130762	0.99046141	0.98957610	0.98865175	0.98768836	0.98668593	0.98564458	0.98456436	0.98344523	0.98228723	0.98109055	0.97985506	0.97858089	0.97726810	0.97591674	0.97452688	0.97309852	0.97163171	0.97012657	0.96858317	0.96700150	0.96538162	0.96372366	0.96202767	0.96029371	0.95852178	0.95671207	0.95486456	0.95297933	0.95105654	0.94909614	0.94709831	0.94506305	0.94299054	0.94088078	0.93873388	0.93654990	0.93432891	0.93207109	0.92977649	0.92744517	0.92507720	0.92267275	0.92023182	0.91775465	0.91524118	0.91269159	0.91010594	0.90748441	0.90482706	0.90213394	0.89940524	0.89664102	0.89384145	0.89100653	0.88813645	0.88523132	0.88229120	0.87931633	0.87630665	0.87326247	0.87018377	0.86707067	0.86392343	0.86074203	0.85752666	0.85427743	0.85099447	0.84767795	0.84432793	0.84094459	0.83752805	0.83407843	0.83059591	0.82708055	0.82353258	0.81995213	0.81633925	0.81269419	0.80901700	0.80530787	0.80156696	0.79779446	0.79399037	0.79015499	0.78628844	0.78239083	0.77846229	0.77450305	0.77051324	0.76649302	0.76244253	0.75836194	0.75425136	0.75011104	0.74594116	0.74174178	0.73751312	0.73325533	0.72896862	0.72465312	0.72030902	0.71593648	0.71153569	0.70710677	0.70264995	0.69816542	0.69365329	0.68911380	0.68454713	0.67995340	0.67533278	0.67068559	0.66601187	0.66131186	0.65658575	0.65183371	0.64705598	0.64225262	0.63742399	0.63257015	0.62769139	0.62278777	0.61785960	0.61290705	0.60793030	0.60292953	0.59790498	0.59285682	0.58778524	0.58269048	0.57757270	0.57243210	0.56726897	0.56208336	0.55687565	0.55164587	0.54639435	0.54112124	0.53582680	0.53051120	0.52517462	0.51981735	0.51443952	0.50904143	0.50362319	0.49818510	0.49272734	0.48725012	0.48175368	0.47623819	0.47070393	0.46515107	0.45957986	0.45399049	0.44838321	0.44275823	0.43711576	0.43145606	0.42577928	0.42008573	0.41437557	0.40864909	0.40290645	0.39714789	0.39137366	0.38558400	0.37977910	0.37395921	0.36812454	0.36227536	0.35641187	0.35053432	0.34464294	0.33873793	0.33281955	0.32688802	0.32094362	0.31498653	0.30901700	0.30303526	0.29704159	0.29103616	0.28501925	0.27899110	0.27295193	0.26690200	0.26084152	0.25477073	0.24868989	0.24259923	0.23649900	0.23038943	0.22427076	0.21814324	0.21200711	0.20586261	0.19970998	0.19354947	0.18738131	0.18120576	0.17502306	0.16883345	0.16263716	0.15643446	0.15022559	0.14401078	0.13779029	0.13156436	0.12533323	0.11909716	0.11285639	0.10661115	0.10036171	0.094108313	0.087851197	0.081590615	0.075326808	0.069060028	0.062790520	0.056518536	0.050244316	0.043968119	0.037690181	0.031410757	0.025130095	0.018848440	0.012566040	0.0062831440	-3.2162452e-16	-0.0062831440	-0.012566040	-0.018848440	-0.025130095	-0.031410757	-0.037690181	-0.043968119	-0.050244316	-0.056518536	-0.062790520	-0.069060028	-0.075326808	-0.081590615	-0.087851197	-0.094108313	-0.10036171	-0.10661115	-0.11285639	-0.11909716	-0.12533323	-0.13156436	-0.13779029	-0.14401078	-0.15022559	-0.15643446	-0.16263716	-0.16883345	-0.17502306	-0.18120576	-0.18738131	-0.19354947	-0.19970998	-0.20586261	-0.21200711	-0.21814324	-0.22427076	-0.23038943	-0.23649900	-0.24259923	-0.24868989	-0.25477073	-0.26084152	-0.26690200	-0.27295193	-0.27899110	-0.28501925	-0.29103616	-0.29704159	-0.30303526	-0.30901700	-0.31498653	-0.32094362	-0.32688802	-0.33281955	-0.33873793	-0.34464294	-0.35053432	-0.35641187	-0.36227536	-0.36812454	-0.37395921	-0.37977910	-0.38558400	-0.39137366	-0.39714789	-0.40290645	-0.40864909	-0.41437557	-0.42008573	-0.42577928	-0.43145606	-0.43711576	-0.44275823	-0.44838321	-0.45399049	-0.45957986	-0.46515107	-0.47070393	-0.47623819	-0.48175368	-0.48725012	-0.49272734	-0.49818510	-0.50362319	-0.50904143	-0.51443952	-0.51981735	-0.52517462	-0.53051120	-0.53582680	-0.54112124	-0.54639435	-0.55164587	-0.55687565	-0.56208336	-0.56726897	-0.57243210	-0.57757270	-0.58269048	-0.58778524	-0.59285682	-0.59790498	-0.60292953	-0.60793030	-0.61290705	-0.61785960	-0.62278777	-0.62769139	-0.63257015	-0.63742399	-0.64225262	-0.64705598	-0.65183371	-0.65658575	-0.66131186	-0.66601187	-0.67068559	-0.67533278	-0.67995340	-0.68454713	-0.68911380	-0.69365329	-0.69816542	-0.70264995	-0.70710677	-0.71153569	-0.71593648	-0.72030902	-0.72465312	-0.72896862	-0.73325533	-0.73751312	-0.74174178	-0.74594116	-0.75011104	-0.75425136	-0.75836194	-0.76244253	-0.76649302	-0.77051324	-0.77450305	-0.77846229	-0.78239083	-0.78628844	-0.79015499	-0.79399037	-0.79779446	-0.80156696	-0.80530787	-0.80901700	-0.81269419	-0.81633925	-0.81995213	-0.82353258	-0.82708055	-0.83059591	-0.83407843	-0.83752805	-0.84094459	-0.84432793	-0.84767795	-0.85099447	-0.85427743	-0.85752666	-0.86074203	-0.86392343	-0.86707067	-0.87018377	-0.87326247	-0.87630665	-0.87931633	-0.88229120	-0.88523132	-0.88813645	-0.89100653	-0.89384145	-0.89664102	-0.89940524	-0.90213394	-0.90482706	-0.90748441	-0.91010594	-0.91269159	-0.91524118	-0.91775465	-0.92023182	-0.92267275	-0.92507720	-0.92744517	-0.92977649	-0.93207109	-0.93432891	-0.93654990	-0.93873388	-0.94088078	-0.94299054	-0.94506305	-0.94709831	-0.94909614	-0.95105654	-0.95297933	-0.95486456	-0.95671207	-0.95852178	-0.96029371	-0.96202767	-0.96372366	-0.96538162	-0.96700150	-0.96858317	-0.97012657	-0.97163171	-0.97309852	-0.97452688	-0.97591674	-0.97726810	-0.97858089	-0.97985506	-0.98109055	-0.98228723	-0.98344523	-0.98456436	-0.98564458	-0.98668593	-0.98768836	-0.98865175	-0.98957610	-0.99046141	-0.99130762	-0.99211472	-0.99288261	-0.99361134	-0.99430078	-0.99495101	-0.99556196	-0.99613363	-0.99666595	-0.99715889	-0.99761254	-0.99802673	-0.99840152	-0.99873698	-0.99903291	-0.99928945	-0.99950653	-0.99968421	-0.99982238	-0.99992102	-0.99998027	-1	-0.99998027	-0.99992102	-0.99982238	-0.99968421	-0.99950653	-0.99928945	-0.99903291	-0.99873698	-0.99840152	-0.99802673	-0.99761254	-0.99715889	-0.99666595	-0.99613363	-0.99556196	-0.99495101	-0.99430078	-0.99361134	-0.99288261	-0.99211472	-0.99130762	-0.99046141	-0.98957610	-0.98865175	-0.98768836	-0.98668593	-0.98564458	-0.98456436	-0.98344523	-0.98228723	-0.98109055	-0.97985506	-0.97858089	-0.97726810	-0.97591674	-0.97452688	-0.97309852	-0.97163171	-0.97012657	-0.96858317	-0.96700150	-0.96538162	-0.96372366	-0.96202767	-0.96029371	-0.95852178	-0.95671207	-0.95486456	-0.95297933	-0.95105654	-0.94909614	-0.94709831	-0.94506305	-0.94299054	-0.94088078	-0.93873388	-0.93654990	-0.93432891	-0.93207109	-0.92977649	-0.92744517	-0.92507720	-0.92267275	-0.92023182	-0.91775465	-0.91524118	-0.91269159	-0.91010594	-0.90748441	-0.90482706	-0.90213394	-0.89940524	-0.89664102	-0.89384145	-0.89100653	-0.88813645	-0.88523132	-0.88229120	-0.87931633	-0.87630665	-0.87326247	-0.87018377	-0.86707067	-0.86392343	-0.86074203	-0.85752666	-0.85427743	-0.85099447	-0.84767795	-0.84432793	-0.84094459	-0.83752805	-0.83407843	-0.83059591	-0.82708055	-0.82353258	-0.81995213	-0.81633925	-0.81269419	-0.80901700	-0.80530787	-0.80156696	-0.79779446	-0.79399037	-0.79015499	-0.78628844	-0.78239083	-0.77846229	-0.77450305	-0.77051324	-0.76649302	-0.76244253	-0.75836194	-0.75425136	-0.75011104	-0.74594116	-0.74174178	-0.73751312	-0.73325533	-0.72896862	-0.72465312	-0.72030902	-0.71593648	-0.71153569	-0.70710677	-0.70264995	-0.69816542	-0.69365329	-0.68911380	-0.68454713	-0.67995340	-0.67533278	-0.67068559	-0.66601187	-0.66131186	-0.65658575	-0.65183371	-0.64705598	-0.64225262	-0.63742399	-0.63257015	-0.62769139	-0.62278777	-0.61785960	-0.61290705	-0.60793030	-0.60292953	-0.59790498	-0.59285682	-0.58778524	-0.58269048	-0.57757270	-0.57243210	-0.56726897	-0.56208336	-0.55687565	-0.55164587	-0.54639435	-0.54112124	-0.53582680	-0.53051120	-0.52517462	-0.51981735	-0.51443952	-0.50904143	-0.50362319	-0.49818510	-0.49272734	-0.48725012	-0.48175368	-0.47623819	-0.47070393	-0.46515107	-0.45957986	-0.45399049	-0.44838321	-0.44275823	-0.43711576	-0.43145606	-0.42577928	-0.42008573	-0.41437557	-0.40864909	-0.40290645	-0.39714789	-0.39137366	-0.38558400	-0.37977910	-0.37395921	-0.36812454	-0.36227536	-0.35641187	-0.35053432	-0.34464294	-0.33873793	-0.33281955	-0.32688802	-0.32094362	-0.31498653	-0.30901700	-0.30303526	-0.29704159	-0.29103616	-0.28501925	-0.27899110	-0.27295193	-0.26690200	-0.26084152	-0.25477073	-0.24868989	-0.24259923	-0.23649900	-0.23038943	-0.22427076	-0.21814324	-0.21200711	-0.20586261	-0.19970998	-0.19354947	-0.18738131	-0.18120576	-0.17502306	-0.16883345	-0.16263716	-0.15643446	-0.15022559	-0.14401078	-0.13779029	-0.13156436	-0.12533323	-0.11909716	-0.11285639	-0.10661115	-0.10036171	-0.094108313	-0.087851197	-0.081590615	-0.075326808	-0.069060028	-0.062790520	-0.056518536	-0.050244316	-0.043968119	-0.037690181	-0.031410757	-0.025130095	-0.018848440	-0.012566040	-0.0062831440];
        flag = 1;
        add = 1;
    else
        flag = 1;
    end
    
    if(add < 1000)
        add = add + 1;
    else
        add = 1;
    end

    SINE_OUT = single(SINE(add));

end

== matlab function Asw_DCAC/Unipolar fast and slow modulation ==
  data: SIN input single; Top_High_Frequency output single; Bottom_High_Frequency output single; Low_Frequency output single
function [Top_High_Frequency, Bottom_High_Frequency, Low_Frequency]  = SPWM(SIN)
    
    Top_High_Frequency = single(0);
    Bottom_High_Frequency = single(0);
    Low_Frequency = single(0);

    if (SIN >= 0)
        Top_High_Frequency = single(SIN);
        Low_Frequency = single(0);
    else 
        Bottom_High_Frequency = -single(SIN);
        Low_Frequency = single(1);
    end
end
